simulink model "GS_model"  (R2018b)
settings: Solver=ode5  StartTime=0.0  StopTime=SimuStopTime  FixedStep=T_Simu  RelTol=1e-3
InitFcn:
  | Initial
undefined symbols (not defined in the file or in its folder): Aba10, Aba20, aeroCIP2006_S, aeroCIP2006_X, aeroCIP2006_Y, Agl0, Ass_kS, Ass_n1, Ass_n2, Ass_n3, Ass_n4, Ass_Noise, Ass_R, Ass_Resolution, Ass_TmOrder, AssA_Fix_Abs, AssB_Fix_Abs, AssC_Fix_Abs, AssD_Fix_Abs, AssE_Fix_Aps, AssF_Fix_Aps, C, c_max, c_min, Cd, CenterOfFigNX, CenterOfFigNY, CenterOfFigNZ, CenterOfFigP1, CenterOfFigP2, CenterOfFigPX, CenterOfFigPY, CenterOfFigPZ, Cmu, Crou, DEG2RAD, DiscIntNeverNeededParam, Eg_Dir, Eg_F, Eg_PrepareTime, Eg_r_L_L, Fw_Abf, Fw_Hmax, Fw_J, Fw_Spd0, Fw_Tmax, git_hash_BaseLine, git_hash_Project, Gnss_Noise_Pos, Gnss_Noise_Vel, Gnss_PropgationTime, GyroA_Fix_Abg, GyroA_Noise, GyroB_Fix_Abg, GyroB_Noise, GyroC_Fix_Abg, GyroC_Noise, GyroD_Fix_Abg, GyroD_Noise, h ... (+94)
libraries: simulink x308, sharedutil x46, aerolibutil x37, sharedtransform x31, vrlib x14, aerolibgravity2 x2
(part 20 of 20)

== matlab function GS_model/Subsystem2/Subsystem/PhysicsModel/Subsystem3/Subsystem1/MATLAB Function2 ==
  data: Agl input; A output; Order input
function A = Agl2DCM(Agl,Order)
% 输入：(1)转序，123或213等
%      (2)转角，按照转序顺序排列，如312转序角度顺序为[zxy];
A = eye(3);
Num = size(Agl,1);
for i = 1:Num
    if Order(i) == 1
        A1 = Rx(Agl(i));
    elseif Order(i) == 2
        A1 = Ry(Agl(i));
    else
        A1 = Rz(Agl(i));
    end
    A = A1*A;
end
end
function A = Rx(alpha)
A = [1 0 0;0 cos(alpha) sin(alpha);0 -sin(alpha) cos(alpha)];
end
function A = Ry(alpha)
A = [cos(alpha) 0 -sin(alpha);0 1 0;sin(alpha) 0 cos(alpha)];
end
function A = Rz(alpha)
A = [cos(alpha) sin(alpha) 0;-sin(alpha) cos(alpha) 0;0 0 1];
end

== matlab function GS_model/Subsystem2/Subsystem/PhysicsModel/Subsystem3/Subsystem1/MATLAB Function3 ==
  data: Agl input; A output; Order input
function A = Agl2DCM(Agl,Order)
% 输入：(1)转序，123或213等
%      (2)转角，按照转序顺序排列，如312转序角度顺序为[zxy];
A = eye(3);
Num = size(Agl,1);
for i = 1:Num
    if Order(i) == 1
        A1 = Rx(Agl(i));
    elseif Order(i) == 2
        A1 = Ry(Agl(i));
    else
        A1 = Rz(Agl(i));
    end
    A = A1*A;
end
end
function A = Rx(alpha)
A = [1 0 0;0 cos(alpha) sin(alpha);0 -sin(alpha) cos(alpha)];
end
function A = Ry(alpha)
A = [cos(alpha) 0 -sin(alpha);0 1 0;sin(alpha) 0 cos(alpha)];
end
function A = Rz(alpha)
A = [cos(alpha) sin(alpha) 0;-sin(alpha) cos(alpha) 0;0 0 1];
end
